simulink model "Watermark_Linear"  (R2021a)
settings: Solver=VariableStepAuto  StartTime=0.0  StopTime=tsim  RelTol=1e-3
undefined symbols (not defined in the file): Adlin, Adlin_un, Bdlin, Bdlin_un, C, Cdlin, K, L, m, n, rlin0, seuil_H0, sigma2_b, SigmaInv, Ts, W
libraries: dspsrcs4 x6, simulink x3, commfilt2 x1
settings Model: Creator=aperodou  LastModifiedBy=Arthur
settings SolverCC: AlgebraicLoopSolver=TrustRegion
settings DebuggingCC: SFMachineParentedDataDiag=warning

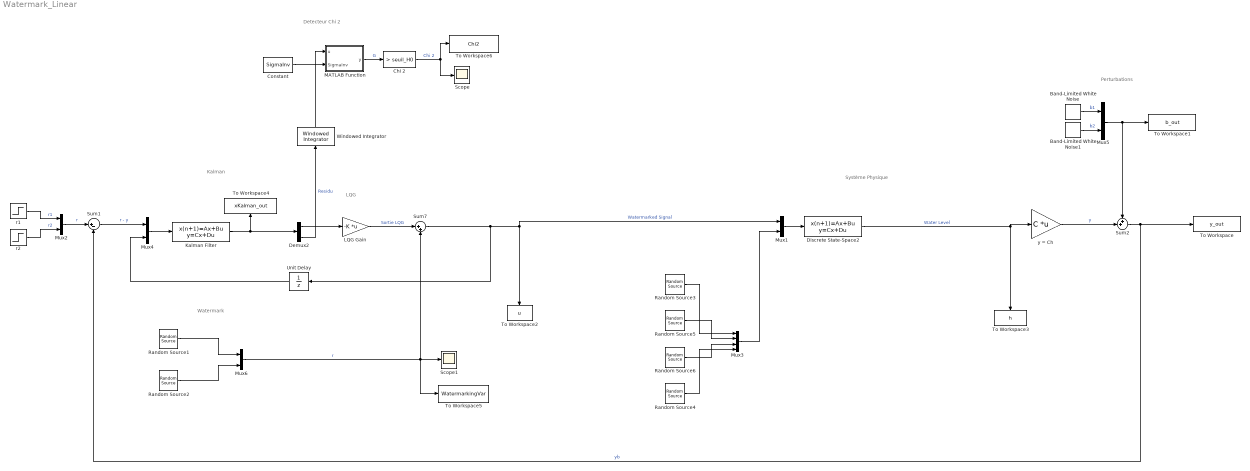
== system Watermark_Linear ==
  note: Kalman
  note: Perturbations
  note: Système Physique
  note: Detecteur Chi 2
  note: LQG
  note: Watermark
  Band-Limited White Noise : simulink/Sources/Band-Limited White Noise  Cov=[ sigma2_b ]  Ts=Ts  seed=[23341]
  Band-Limited White Noise1 : simulink/Sources/Band-Limited White Noise  Cov=[ sigma2_b]  Ts=Ts  seed=[20000]
  Chi 2 : simulink/Logic and Bit Operations/Compare To Constant  relop=>  const=seuil_H0  OutDataTypeStr=boolean
  Constant : Constant  Value=SigmaInv
  Demux2 : Demux  Outputs=2
  Discrete State-Space2 : DiscreteStateSpace  A=Adlin_un  B=Bdlin_un  C=eye(n)  D=zeros(n, n+m)  InitialCondition=zeros(n,1)  SampleTime=Ts
  Kalman Filter : DiscreteStateSpace  A=Adlin  B=[zeros(n,m) -Bdlin]  C=[eye(n) - L*Cdlin ; -Cdlin]  D=[L zeros(n,m) ; eye(m) zeros(m,m)]  InitialCondition=zeros(n,1)  SampleTime=Ts
  LQG Gain : Gain  Gain=-K  Multiplication=Matrix(K*u) (u vector)
  MATLAB Function : MATLAB Function  TreatAsAtomicUnit=on
  Mux{1..2,4..6} (5 alike) : Mux  Inputs=2
  Mux3 : Mux
  Random Source1 : dspsrcs4/Random Source  SrcType=Gaussian  NormMethod=Ziggurat  CltLength=12  MinVal=0  MaxVal=1  MeanVal=0  VarVal=varW  RepMode=Not repeatable  rawSeed=1  IsInherit=off  SampMode=Discrete  SampTime=1  SampFrame=1  DataType=Double  OutComplex=Real  OutputFrames=off
  Random Source2 : dspsrcs4/Random Source  SrcType=Gaussian  NormMethod=Ziggurat  CltLength=12  MinVal=0  MaxVal=1  MeanVal=0  VarVal=varW  RepMode=Not repeatable  rawSeed=1  IsInherit=off  SampMode=Discrete  SampTime=1  SampFrame=1  DataType=Double  OutComplex=Real  OutputFrames=off
  Random Source3 : dspsrcs4/Random Source  SrcType=Gaussian  NormMethod=Ziggurat  CltLength=12  MinVal=0  MaxVal=1  MeanVal=0  VarVal=W(1,1)  RepMode=Not repeatable  rawSeed=1  IsInherit=off  SampMode=Continuous  SampTime=1  SampFrame=1  DataType=Double  OutComplex=Real  OutputFrames=off
  Random Source4 : dspsrcs4/Random Source  SrcType=Gaussian  NormMethod=Ziggurat  CltLength=12  MinVal=0  MaxVal=1  MeanVal=0  VarVal=W(4,4)  RepMode=Not repeatable  rawSeed=1  IsInherit=off  SampMode=Discrete  SampTime=1  SampFrame=1  DataType=Double  OutComplex=Real  OutputFrames=off
  Random Source5 : dspsrcs4/Random Source  SrcType=Gaussian  NormMethod=Ziggurat  CltLength=12  MinVal=0  MaxVal=1  MeanVal=0  VarVal=W(2,2)  RepMode=Not repeatable  rawSeed=1  IsInherit=off  SampMode=Discrete  SampTime=1  SampFrame=1  DataType=Double  OutComplex=Real  OutputFrames=off
  Random Source6 : dspsrcs4/Random Source  SrcType=Gaussian  NormMethod=Ziggurat  CltLength=12  MinVal=0  MaxVal=1  MeanVal=0  VarVal=W(3,3)  RepMode=Not repeatable  rawSeed=1  IsInherit=off  SampMode=Discrete  SampTime=1  SampFrame=1  DataType=Double  OutComplex=Real  OutputFrames=off
  Scope : Scope
  Scope1 : Scope
  Sum1 : Sum  Inputs=|+-  SaturateOnIntegerOverflow=on
  Sum2 : Sum  Inputs=++|  SaturateOnIntegerOverflow=on
  Sum7 : Sum  Inputs=|++  SaturateOnIntegerOverflow=on
  To Workspace : ToWorkspace  VariableName=y_out  SaveFormat=Timeseries  SampleTime=-1
  To Workspace1 : ToWorkspace  VariableName=b_out  SaveFormat=Timeseries  SampleTime=-1
  To Workspace2 : ToWorkspace  VariableName=u  SampleTime=-1
  To Workspace3 : ToWorkspace  VariableName=h  SampleTime=-1
  To Workspace4 : ToWorkspace  VariableName=xKalman_out  SaveFormat=Timeseries  SampleTime=-1
  To Workspace5 : ToWorkspace  VariableName=WatermarkingVar  SaveFormat=Timeseries  SampleTime=-1
  To Workspace6 : ToWorkspace  VariableName=Chi2  SampleTime=-1
  Unit Delay : UnitDelay  SampleTime=Ts  HasFrameUpgradeWarning=on
  Windowed Integrator : commfilt2/Windowed Integrator  integperiod=timeWindow  roundingMode=Floor  overflowMode=off  coeffDataTypeStr=Inherit: Same word length as input  coeffMin=[]  coeffMax=[]  coeffLastDataTypeStr=Inherit: Same word length as input  accumDataTypeStr=Inherit: Same as product output  accumLastDataTypeStr=Inherit: Same as product output  outputDataTypeStr=Inherit: Same as accumulator  outputMin=[]  outputMax=[]  outputLastDataTypeStr=Inherit: Same as accumulator
      settings: SourceProductBaseCode=CM
  r1 : Step  Time=0  After=rlin0(1)  SampleTime=0
  r2 : Step  Time=0  After=rlin0(2)  SampleTime=0
  y = Ch : Gain  Gain=C  Multiplication=Matrix(K*u) (u vector)
  wires:
  Discrete State-Space2/1 -> y = Ch/1, To Workspace3/1  "Water Level"
  Mux2/1 -> Sum1/1  "r"
  Sum2/1 -> Sum1/2, To Workspace/1  "yb"
  y = Ch/1 -> Sum2/2  "y"
  r2/1 -> Mux2/2  "r2"
  r1/1 -> Mux2/1  "r1"
  Kalman Filter/1 -> Demux2/1, To Workspace4/1
  LQG Gain/1 -> Sum7/1  "Sortie LQG"
  Mux4/1 -> Kalman Filter/1
  Sum1/1 -> Mux4/1  "r - y"
  Unit Delay/1 -> Mux4/2
  Band-Limited White Noise/1 -> Mux5/1  "b1"
  Band-Limited White Noise1/1 -> Mux5/2  "b2"
  Mux5/1 -> Sum2/1, To Workspace1/1
  Demux2/1 -> LQG Gain/1
  Constant/1 -> MATLAB Function/2(SigmaInv)
  MATLAB Function/1(y) -> Chi 2/1  "G"
  Demux2/2 -> Windowed Integrator/1  "Residu"
  Chi 2/1 -> To Workspace6/1, Scope/1  "Chi 2"
  Random Source1/1 -> Mux6/1
  Mux6/1 -> To Workspace5/1, Sum7/2, Scope1/1  "r"
  Random Source2/1 -> Mux6/2
  Sum7/1 -> To Workspace2/1, Mux1/1, Unit Delay/1  "Watermarked Signal"
  Windowed Integrator/1 -> MATLAB Function/1(u)
  Mux3/1 -> Mux1/2
  Mux1/1 -> Discrete State-Space2/1
  Random Source3/1 -> Mux3/1
  Random Source4/1 -> Mux3/4
  Random Source6/1 -> Mux3/3
  Random Source5/1 -> Mux3/2

== matlab function Watermark_Linear/MATLAB Function ==
  data: u input; y output; SigmaInv input
function y = fcn(u,SigmaInv)

y = u'*SigmaInv*u;

end
